simulink model "LP8_orig"  (R2019a)
settings: Solver=FixedStepDiscrete  StartTime=0.0  StopTime=stop_time  RelTol=1e-3
InitFcn:
  | sm_callback_init
StopFcn:
  | sm_callback_stop
undefined symbols (not defined in the file or in its folder): dfilt, mp
libraries: simulink x3, dsparch4 x1
settings Model: Creator=Ross  LastModifiedBy=Ross
settings DataIOCC: ReturnWorkspaceOutputs=off
settings OptimizationCC: BlockReduction=off  ConditionallyExecuteInputs=off  DefaultParameterBehavior=Inlined
settings DebuggingCC: ReadBeforeWriteMsg=DisableAll  WriteAfterWriteMsg=DisableAll  WriteAfterReadMsg=DisableAll  AlgebraicLoopMsg=error  MultiTaskDSMMsg=none  SingleTaskRateTransMsg=error  PregeneratedLibrarySubsystemCodeDiagnostic=none  ArithmeticOperatorsInVariantConditions=warning
settings HardwareCC: ProdBitPerPointer=32  ProdBitPerSizeT=32  ProdBitPerPtrDiffT=32  ProdLargestAtomicFloat=None  ProdIntDivRoundTo=Undefined  ProdEndianess=Unspecified  ProdWordSize=32  ProdHWDeviceType=ASIC/FPGA->ASIC/FPGA  TargetBitPerPointer=64  TargetBitPerSizeT=64  TargetBitPerPtrDiffT=64  TargetLongLongMode=on  TargetIntDivRoundTo=Zero  TargetEndianess=LittleEndian  TargetWordSize=64  TargetHWDeviceType=Custom Processor->MATLAB Host Computer  ProdEqTarget=off
settings ModelReferenceCC: UpdateModelReferenceTargets=IfOutOfDate
settings SFSimCC: SFSimEcho=off  SimUseLocalCustomCode=off
settings RTWCC: RTWUseLocalCustomCode=off

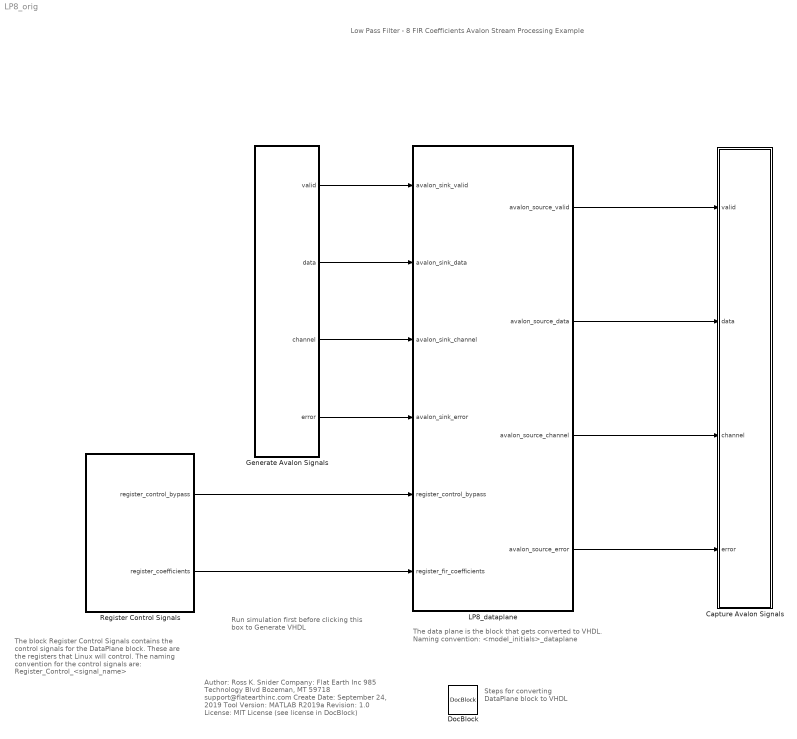
== system LP8_orig ==
  note: The data plane is the block that gets converted to VHDL. Naming convention: <model_initials>_dataplane
  note: Author:          Ross K. Snider
      | Company:     Flat Earth Inc
      |                       985 Technology Blvd
      |                       Bozeman, MT 59718
      |                       support@flatearthinc.com
      | Create Date:  September 24, 2019
      | Tool Version:  MATLAB R2019a
      | Revision:        1.0
      | License:          MIT License (see license in DocBlock)
  note: Steps for converting
      | DataPlane block
      | to VHDL
  note: Low Pass Filter - 8 FIR Coefficients
      | Avalon Stream Processing Example
  note: Run simulation first
      | before clicking this box to
      | Generate VHDL
  note: The block Register Control Signals contains
      | the control signals for the DataPlane block.
      | These are the registers that Linux will control.
      | The naming convention for the control
      | signals are:  Register_Control_<signal_name>
  Capture Avalon Signals : Subsystem
  DocBlock : simulink/Model-Wide Utilities/DocBlock  DocumentType=HTML
  Generate Avalon Signals : Subsystem
  LP8_dataplane : Subsystem  TreatAsAtomicUnit=on
  Register Control Signals : Subsystem
  wires:
  Generate Avalon Signals/2(data) -> LP8_dataplane/2(avalon_sink_data)
  Generate Avalon Signals/1(valid) -> LP8_dataplane/1(avalon_sink_valid)
  Generate Avalon Signals/3(channel) -> LP8_dataplane/3(avalon_sink_channel)
  Generate Avalon Signals/4(error) -> LP8_dataplane/4(avalon_sink_error)
  LP8_dataplane/2(avalon_source_data) -> Capture Avalon Signals/2(data)
  LP8_dataplane/1(avalon_source_valid) -> Capture Avalon Signals/1(valid)
  LP8_dataplane/3(avalon_source_channel) -> Capture Avalon Signals/3(channel)
  LP8_dataplane/4(avalon_source_error) -> Capture Avalon Signals/4(error)
  Register Control Signals/2(register_coefficients) -> LP8_dataplane/6(register_fir_coefficients)
  Register Control Signals/1(register_control_bypass) -> LP8_dataplane/5(register_control_bypass)

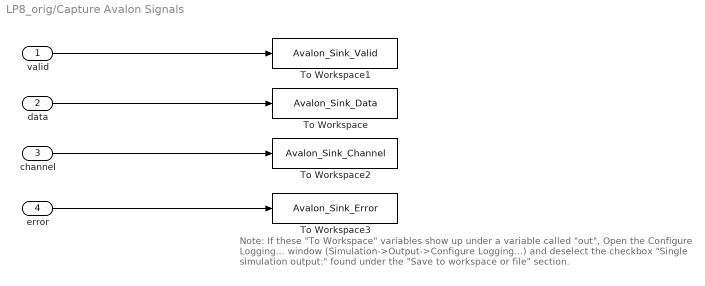
== system LP8_orig/Capture Avalon Signals ==
  note: Note:  If these "To Workspace" variables show up under a variable called "out",
      | Open the Configure Logging... window (Simulation->Output->Configure Logging...)
      | and deselect the checkbox "Single simulation output:" found under the "Save to workspace or file" section.
  valid : Inport
  data : Inport  Port=2
  channel : Inport  Port=3
  error : Inport  Port=4
  To Workspace : ToWorkspace  VariableName=Avalon_Sink_Data  SaveFormat=Timeseries  SampleTime=-1
  To Workspace1 : ToWorkspace  VariableName=Avalon_Sink_Valid  SaveFormat=Timeseries  SampleTime=-1
  To Workspace2 : ToWorkspace  VariableName=Avalon_Sink_Channel  SaveFormat=Timeseries  SampleTime=-1
  To Workspace3 : ToWorkspace  VariableName=Avalon_Sink_Error  SaveFormat=Timeseries  SampleTime=-1
  wires:
  data/1 -> To Workspace/1
  valid/1 -> To Workspace1/1
  error/1 -> To Workspace3/1
  channel/1 -> To Workspace2/1

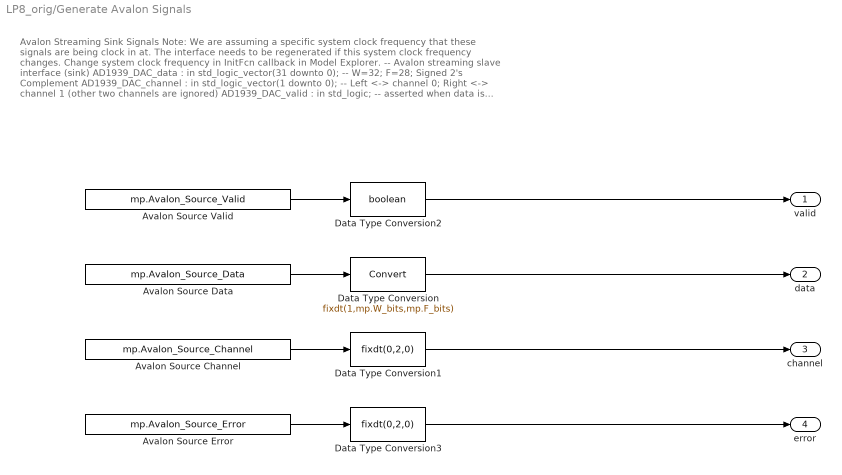
== system LP8_orig/Generate Avalon Signals ==
  note: Avalon Streaming Sink Signals
      | Note: We are assuming a specific system clock frequency that these signals are being clock in at.
      | The interface needs to be regenerated if this system clock frequency changes. Change system clock frequency in InitFcn callback in Model Explorer.
      |
      | -- Avalon streaming slave interface (sink)
      | AD1939_DAC_data : in std_logic_vector(31 downto 0); -- W=32; F=28; Signed 2's Complement
      | AD1939_DAC_channel : in std_logic_vector(1 downto 0); -- Left <-> channel 0; Right <-> channel 1 (other two channels are ignored)
      | AD1939_DAC_valid : in std_logic; -- asserted when data is valid
      | AD1939_DAC_error : in std_logic_vector(1 downto 0) -- error channel is ignored, assumed to be error free at this point
      |
      | For more information on the data-channel-valid protocol, s ee chapter 5 in Intel's Avalon Interfaced Specification (p. 40) at https://www.intel.com/content/dam/www/programmable/us/en/pdfs/literature/manual/mnl_avalon_spec.pdf
  Avalon Source Channel : FromWorkspace  VariableName=mp.Avalon_Source_Channel  OutDataTypeStr=double  SampleTime=mp.Ts_system
  "Avalon Source Data " : FromWorkspace  VariableName=mp.Avalon_Source_Data  OutDataTypeStr=double  SampleTime=mp.Ts_system
  Avalon Source Error : FromWorkspace  VariableName=mp.Avalon_Source_Error  OutDataTypeStr=double  SampleTime=mp.Ts_system
  Avalon Source Valid : FromWorkspace  VariableName=mp.Avalon_Source_Valid  OutDataTypeStr=double  SampleTime=mp.Ts_system
  Data Type Conversion : DataTypeConversion  OutDataTypeStr=fixdt(1,mp.W_bits,mp.F_bits)
  Data Type Conversion1 : DataTypeConversion  OutDataTypeStr=fixdt(0,2,0)
  Data Type Conversion2 : DataTypeConversion  OutDataTypeStr=boolean
  Data Type Conversion3 : DataTypeConversion  OutDataTypeStr=fixdt(0,2,0)
  valid : Outport
  data : Outport  Port=2
  channel : Outport  Port=3
  error : Outport  Port=4
  wires:
  Data Type Conversion1/1 -> channel/1
  Data Type Conversion2/1 -> valid/1
  Avalon Source Error/1 -> Data Type Conversion3/1
  Data Type Conversion/1 -> data/1
  Avalon Source Valid/1 -> Data Type Conversion2/1
  Data Type Conversion3/1 -> error/1
  Avalon Source Channel/1 -> Data Type Conversion1/1
  "Avalon Source Data "/1 -> Data Type Conversion/1

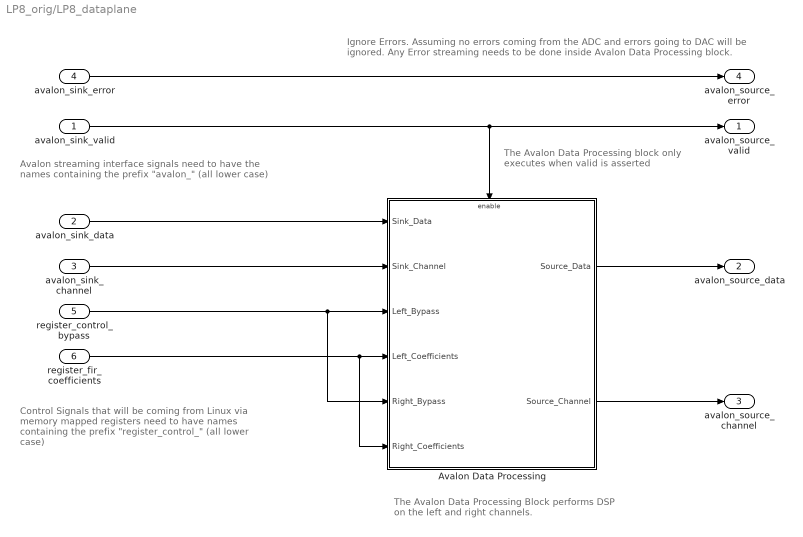
== system LP8_orig/LP8_dataplane ==
  note: Control Signals that will be coming from Linux via
      | memory mapped registers need to have names
      | containing the prefix "register_control_"
      | (all lower case)
  note: The Avalon Data Processing Block
      | performs DSP on the left and right channels.
  note: The Avalon Data Processing block
      | only executes when valid is asserted
  note: Ignore Errors.
      | Assuming no errors coming from the ADC and errors going to DAC will be ignored.
      | Any Error streaming needs to be done inside Avalon Data Processing block.
  note: Avalon streaming interface signals need to have the
      | names containing the prefix "avalon_"
      | (all lower case)
  avalon_sink_valid : Inport
  avalon_sink_data : Inport  Port=2
  avalon_sink_channel : Inport  Port=3
  avalon_sink_error : Inport  Port=4
  register_control_bypass : Inport  Port=5
  register_fir_coefficients : Inport  Port=6
  Avalon Data Processing : Subsystem  TreatAsAtomicUnit=on
  avalon_source_valid : Outport
  avalon_source_data : Outport  Port=2
  avalon_source_channel : Outport  Port=3
  avalon_source_error : Outport  Port=4
  wires:
  avalon_sink_channel/1 -> Avalon Data Processing/2(Sink_Channel)
  avalon_sink_error/1 -> avalon_source_error/1
  Avalon Data Processing/1(Source_Data) -> avalon_source_data/1
  avalon_sink_valid/1 -> avalon_source_valid/1, Avalon Data Processing/Enable
  avalon_sink_data/1 -> Avalon Data Processing/1(Sink_Data)
  Avalon Data Processing/2(Source_Channel) -> avalon_source_channel/1
  register_control_bypass/1 -> Avalon Data Processing/5(Right_Bypass), Avalon Data Processing/3(Left_Bypass)
  register_fir_coefficients/1 -> Avalon Data Processing/6(Right_Coefficients), Avalon Data Processing/4(Left_Coefficients)

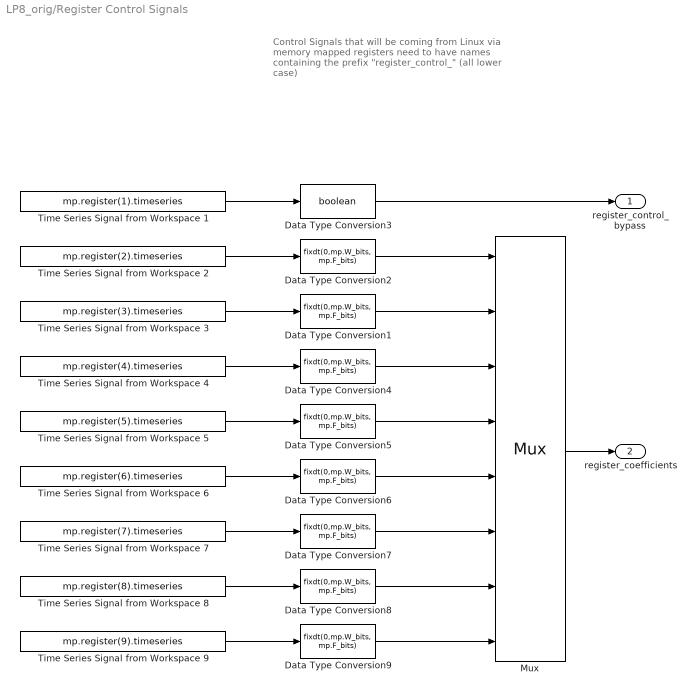
== system LP8_orig/Register Control Signals ==
  note: Control Signals that will be coming from Linux via
      | memory mapped registers need to have names
      | containing the prefix "register_control_"
      | (all lower case)
  Data Type Conversion{1..2,4..9} (8 alike) : DataTypeConversion  OutDataTypeStr=fixdt(0,mp.W_bits, mp.F_bits)
  Data Type Conversion3 : DataTypeConversion  OutDataTypeStr=boolean
  Mux : Mux  Inputs=8
  Time Series Signal from Workspace 1 : FromWorkspace  VariableName=mp.register(1).timeseries  OutDataTypeStr=double  SampleTime=mp.Ts_system
  Time Series Signal from Workspace 2 : FromWorkspace  VariableName=mp.register(2).timeseries  OutDataTypeStr=double  SampleTime=mp.Ts_system
  Time Series Signal from Workspace 3 : FromWorkspace  VariableName=mp.register(3).timeseries  OutDataTypeStr=double  SampleTime=mp.Ts_system
  Time Series Signal from Workspace 4 : FromWorkspace  VariableName=mp.register(4).timeseries  OutDataTypeStr=double  SampleTime=mp.Ts_system
  Time Series Signal from Workspace 5 : FromWorkspace  VariableName=mp.register(5).timeseries  OutDataTypeStr=double  SampleTime=mp.Ts_system
  Time Series Signal from Workspace 6 : FromWorkspace  VariableName=mp.register(6).timeseries  OutDataTypeStr=double  SampleTime=mp.Ts_system
  Time Series Signal from Workspace 7 : FromWorkspace  VariableName=mp.register(7).timeseries  OutDataTypeStr=double  SampleTime=mp.Ts_system
  Time Series Signal from Workspace 8 : FromWorkspace  VariableName=mp.register(8).timeseries  OutDataTypeStr=double  SampleTime=mp.Ts_system
  Time Series Signal from Workspace 9 : FromWorkspace  VariableName=mp.register(9).timeseries  OutDataTypeStr=double  SampleTime=mp.Ts_system
  register_control_bypass : Outport
  register_coefficients : Outport  Port=2
  wires:
  Time Series Signal from Workspace 2/1 -> Data Type Conversion2/1
  Data Type Conversion2/1 -> Mux/1
  Time Series Signal from Workspace 1/1 -> Data Type Conversion3/1
  Data Type Conversion3/1 -> register_control_bypass/1
  Data Type Conversion1/1 -> Mux/2
  Time Series Signal from Workspace 3/1 -> Data Type Conversion1/1
  Data Type Conversion4/1 -> Mux/3
  Time Series Signal from Workspace 4/1 -> Data Type Conversion4/1
  Data Type Conversion5/1 -> Mux/4
  Time Series Signal from Workspace 5/1 -> Data Type Conversion5/1
  Data Type Conversion6/1 -> Mux/5
  Time Series Signal from Workspace 6/1 -> Data Type Conversion6/1
  Data Type Conversion7/1 -> Mux/6
  Time Series Signal from Workspace 7/1 -> Data Type Conversion7/1
  Data Type Conversion8/1 -> Mux/7
  Time Series Signal from Workspace 8/1 -> Data Type Conversion8/1
  Data Type Conversion9/1 -> Mux/8
  Time Series Signal from Workspace 9/1 -> Data Type Conversion9/1
  Mux/1 -> register_coefficients/1

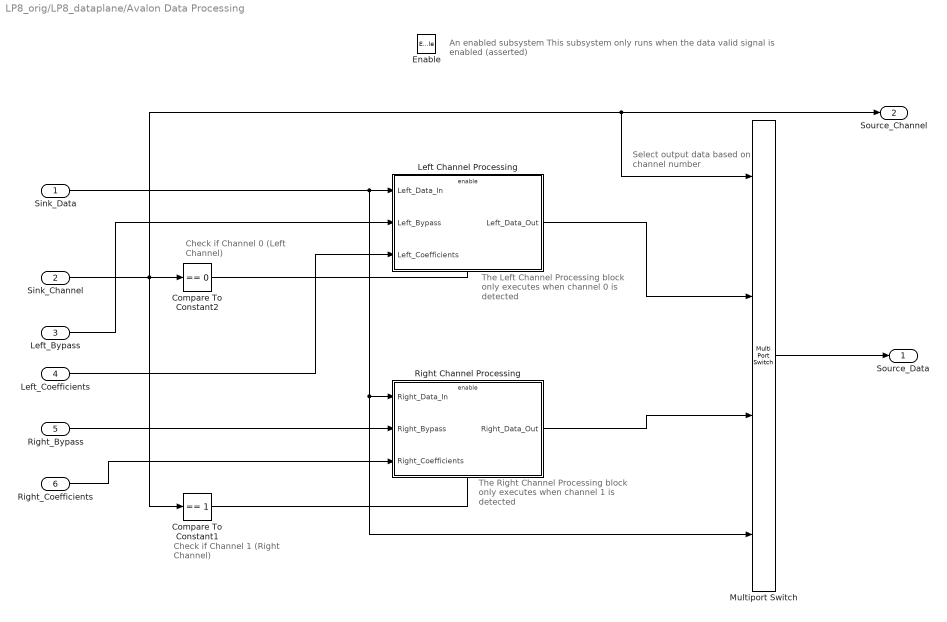
== system LP8_orig/LP8_dataplane/Avalon Data Processing ==
  note: Select output data
      | based on channel number
  note: Check if Channel 0
      | (Left Channel)
  note: The Left Channel Processing block
      | only executes when channel 0
      | is detected
  note: The Right Channel Processing block
      | only executes when channel 1
      | is detected
  note: Check if Channel 1
      | (Right Channel)
  note: An enabled subsystem
      | This subsystem only runs when the data valid signal is enabled (asserted)
  Sink_Data : Inport
  Sink_Channel : Inport  Port=2
  Left_Bypass : Inport  Port=3
  Left_Coefficients : Inport  Port=4
  Right_Bypass : Inport  Port=5
  Right_Coefficients : Inport  Port=6
  Enable : EnablePort
  Compare To Constant1 : simulink/Logic and Bit Operations/Compare To Constant  relop===  const=1  OutDataTypeStr=boolean
  Compare To Constant2 : simulink/Logic and Bit Operations/Compare To Constant  relop===  const=0  OutDataTypeStr=boolean
  Left Channel Processing : Subsystem  TreatAsAtomicUnit=on
  Multiport Switch : MultiPortSwitch  DataPortOrder=Zero-based contiguous  zeroidx=on
  Right Channel Processing : Subsystem  TreatAsAtomicUnit=on
  Source_Data : Outport  InitialOutput=0
  Source_Channel : Outport  Port=2  InitialOutput=0
  wires:
  Sink_Channel/1 -> Source_Channel/1, Multiport Switch/1, Compare To Constant1/1, Compare To Constant2/1
  Compare To Constant2/1 -> Left Channel Processing/Enable
  Compare To Constant1/1 -> Right Channel Processing/Enable
  Sink_Data/1 -> Multiport Switch/4, Right Channel Processing/1(Right_Data_In), Left Channel Processing/1(Left_Data_In)
  Left Channel Processing/1("Left_Data_Out ") -> Multiport Switch/2
  Right Channel Processing/1("Right_Data_Out ") -> Multiport Switch/3
  Multiport Switch/1 -> Source_Data/1
  Left_Bypass/1 -> Left Channel Processing/2(Left_Bypass)
  Right_Bypass/1 -> Right Channel Processing/2(Right_Bypass)
  Left_Coefficients/1 -> Left Channel Processing/3(Left_Coefficients)
  Right_Coefficients/1 -> Right Channel Processing/3(Right_Coefficients)

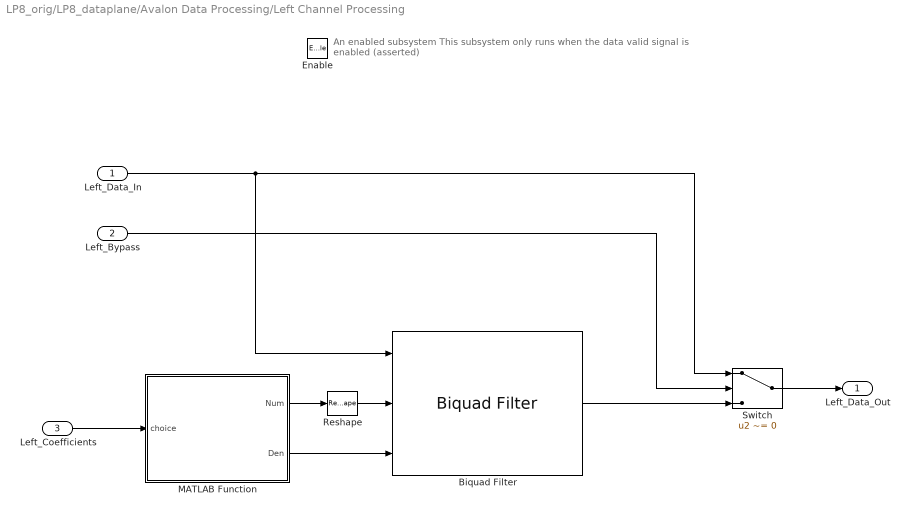
== system LP8_orig/LP8_dataplane/Avalon Data Processing/Left Channel Processing ==
  note: An enabled subsystem
      | This subsystem only runs when the data valid signal is enabled (asserted)
  Left_Data_In : Inport
  Left_Bypass : Inport  Port=2
  Left_Coefficients : Inport  Port=3
  Enable : EnablePort
  Biquad Filter : dsparch4/Biquad Filter  FilterSource=Input port(s)  CoeffSource=Specify via dialog  FilterObject=dfilt.df2tsos([1 0.3 0.4],[1 0.1 0.2])  IIRFiltStruct=Direct form II transposed  BiQuadCoeffs=[1 0.3 0.4 1 0.1 0.2]  ScaleValues=1  IC=0  ICnum=0  ICden=0  a0Flag=Warning  optimizeScaleValues=on  ScaleValueMode=Assume all are unity and optimize  roundingMode=Floor  overflowMode=on  scaleValueFracLength=14  denProdOutputFracLength=30  denAccumFracLength=30  secondMemoryFracLength=15
      settings: SourceProductName=DSP System Toolbox
  MATLAB Function : MATLAB Function  TreatAsAtomicUnit=on
  Reshape : Reshape
  Switch : Switch  Criteria=u2 ~= 0
  "Left_Data_Out " : Outport  InitialOutput=0
  wires:
  Left_Data_In/1 -> Switch/1, Biquad Filter/1
  Biquad Filter/1 -> Switch/3
  Switch/1 -> "Left_Data_Out "/1
  Left_Bypass/1 -> Switch/2
  Left_Coefficients/1 -> MATLAB Function/1(choice)
  MATLAB Function/2(Den) -> Biquad Filter/3
  MATLAB Function/1(Num) -> Reshape/1
  Reshape/1 -> Biquad Filter/2

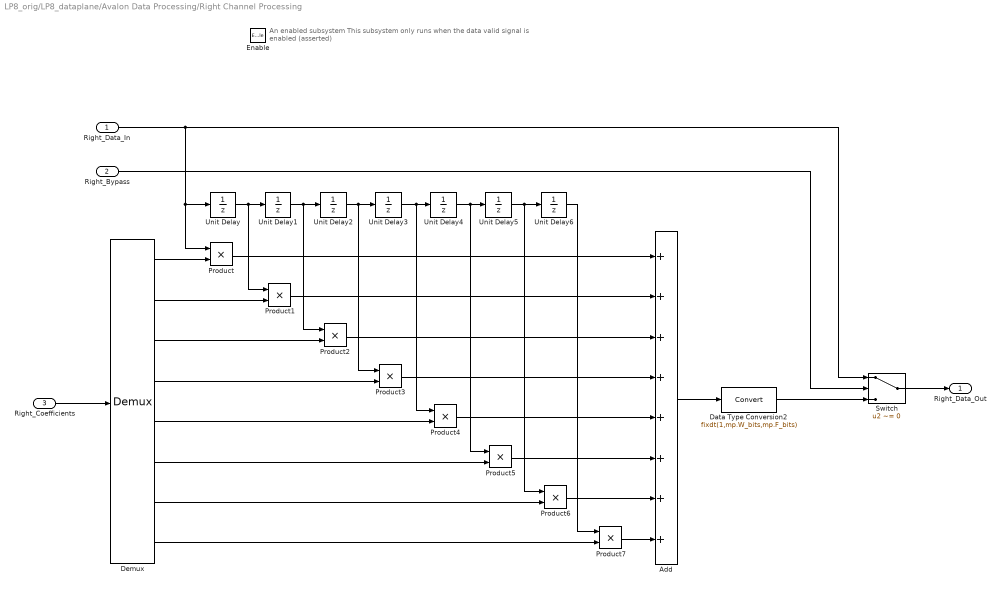
== system LP8_orig/LP8_dataplane/Avalon Data Processing/Right Channel Processing ==
  note: An enabled subsystem
      | This subsystem only runs when the data valid signal is enabled (asserted)
  Right_Data_In : Inport
  Right_Bypass : Inport  Port=2
  Right_Coefficients : Inport  Port=3
  Enable : EnablePort
  Add : Sum  Inputs=++++++++
  Data Type Conversion2 : DataTypeConversion  OutDataTypeStr=fixdt(1,mp.W_bits,mp.F_bits)
  Demux : Demux  Outputs=8
  Product{,1..7} (8 alike) : Product
  Switch : Switch  Criteria=u2 ~= 0
  Unit Delay{,1..6} (7 alike) : UnitDelay  SampleTime=-1  HasFrameUpgradeWarning=on
  "Right_Data_Out " : Outport  InitialOutput=0
  wires:
  Right_Data_In/1 -> Product/1, Unit Delay/1, Switch/1
  Data Type Conversion2/1 -> Switch/3
  Switch/1 -> "Right_Data_Out "/1
  Right_Bypass/1 -> Switch/2
  Unit Delay/1 -> Product1/1, Unit Delay1/1
  Unit Delay1/1 -> Product2/1, Unit Delay2/1
  Unit Delay2/1 -> Product3/1, Unit Delay3/1
  Unit Delay3/1 -> Product4/1, Unit Delay4/1
  Unit Delay4/1 -> Product5/1, Unit Delay5/1
  Unit Delay5/1 -> Product6/1, Unit Delay6/1
  Unit Delay6/1 -> Product7/1
  Product/1 -> Add/1
  Product1/1 -> Add/2
  Product2/1 -> Add/3
  Product3/1 -> Add/4
  Product4/1 -> Add/5
  Product5/1 -> Add/6
  Product6/1 -> Add/7
  Product7/1 -> Add/8
  Add/1 -> Data Type Conversion2/1
  Demux/1 -> Product/2
  Demux/8 -> Product7/2
  Right_Coefficients/1 -> Demux/1
  Demux/2 -> Product1/2
  Demux/3 -> Product2/2
  Demux/4 -> Product3/2
  Demux/5 -> Product4/2
  Demux/6 -> Product5/2
  Demux/7 -> Product6/2

== matlab function LP8_orig/LP8_dataplane/Avalon Data Processing/Left Channel Processing/MATLAB Function ==
  data: choice input; Num output; Den output
function [Num, Den] = fcn(choice)
%#codegen

switch choice
    case 1
        Num = [0.0283    0.0567    0.0283];
        Den = [1.0000   -1.7386    0.8520];
    case 2
        Num = [0.0151    0.0302    0.0151];
        Den = [1.0000   -1.8297    0.8901];
    otherwise
        % do nothing
end
